simulink model "PMSM_braking_regen_and_Eddy_current_using_ABS"  (R2023a)
settings: Solver=VariableStepAuto  StartTime=0.0  StopTime=20  MaxStep=1  RelTol=1e-3
libraries: spsControlledVoltageSourceLib x3, spsVoltageMeasurementLib x3, simulink x2, spsPermanentMagnetSynchronousMachineLib x1, spsThreePhaseSineGeneratorLib x1, sps_lib x1
settings Model: Creator=siddh  LastModifiedBy=siddh

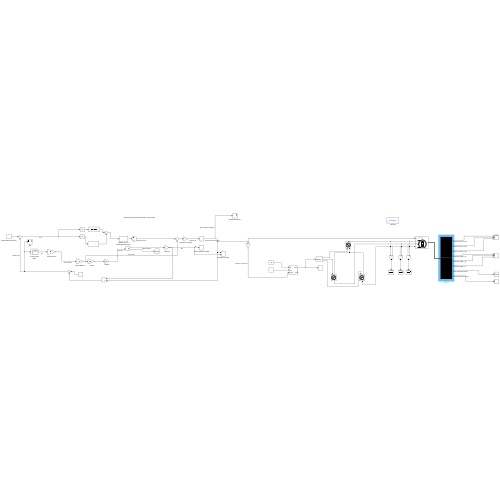
[thumbnail: Simulink's stored preview of the top-level diagram]
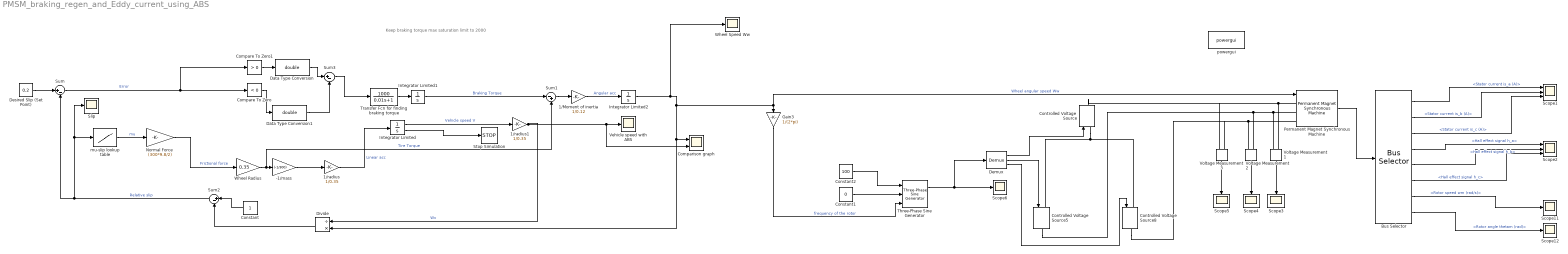
== system PMSM_braking_regen_and_Eddy_current_using_ABS ==
  note: Keep braking torque max saturation limit to 2000
  -1/mass : Gain  Gain=(-1/300)
  1/Moment of inertia : Gain  Gain=1/0.12
  1/radius : Gain  Gain=1/0.35
  1/radius1 : Gain  Gain=1/0.35
  Bus Selector : BusSelector  OutputSignals=Stator current is_a (A),Stator current is_b (A),Stator current is_c (A),Hall effect signal h_a,Hall effect signal h_b,Hall effect signal h_c,Rotor speed wm (rad/s),Rotor angle thetam (rad)
  Compare To Zero : simulink/Logic and Bit Operations/Compare To Zero  relop=<  OutDataTypeStr=boolean
  Compare To Zero1 : simulink/Logic and Bit Operations/Compare To Zero  relop=>  OutDataTypeStr=boolean
  Comparison graph : Scope  NumInputPorts=2
  Constant : Constant
  Constant1 : Constant  Value=0
  Constant2 : Constant  Value=100
  Controlled Voltage Source : spsControlledVoltageSourceLib/Controlled Voltage Source  Initialize=on  Source_Type=AC  Amplitude=100  Phase=0  Frequency=0  Measurements=None
  Controlled Voltage Source5 : spsControlledVoltageSourceLib/Controlled Voltage Source  Initialize=on  Source_Type=AC  Amplitude=0  Phase=0  Frequency=0  Measurements=None
  Controlled Voltage Source8 : spsControlledVoltageSourceLib/Controlled Voltage Source  Initialize=on  Source_Type=AC  Amplitude=0  Phase=0  Frequency=0  Measurements=None
  Data Type Conversion : DataTypeConversion  OutDataTypeStr=double  SaturateOnIntegerOverflow=off
  Data Type Conversion1 : DataTypeConversion  OutDataTypeStr=double  SaturateOnIntegerOverflow=off
  Demux : Demux  Outputs=3
      settings: DisplayOption=none
  "Desired Slip (Set Point) " : Constant  Value=0.2
  Divide : Product  Inputs=/*
  Gain3 : Gain  Gain=1/(2*pi)
  Integrator Limited : Integrator  InitialCondition=30  LimitOutput=on  UpperSaturationLimit=500  LowerSaturationLimit=0  ShowSaturationPort=on
  Integrator Limited1 : Integrator  LimitOutput=on  UpperSaturationLimit=2000  LowerSaturationLimit=0
  Integrator Limited2 : Integrator  InitialCondition=30/0.35  LimitOutput=on  UpperSaturationLimit=500  LowerSaturationLimit=0
  Normal Force : Gain  Gain=(300*9.8/2)
  Permanent Magnet Synchronous Machine : spsPermanentMagnetSynchronousMachineLib/Permanent Magnet Synchronous Machine  NbPhases=3  FluxDistribution=Sinusoidal  RotorType=Round  MechanicalLoad=Speed w  PresetModel=No  ShowDetailedParameters=on  MeasurementBus=off  Resistance=18.7  Inductance=8.5e-3  dqInductances=[8.5e-3,8.5e-3]  La=0.02682  MachineConstant=Flux linkage established by magnets (V.s)  Flux=0.1716  VoltageCst=62.2496  TorqueCst=0.5148  Flat=120  Mechanical=[2.26e-05 1.349e-05 2 0]  PolePairs=2  InitialConditions=[0,0, 0,0]  InitialConditions5ph=[0 0 0 0 0 0]  RefAngle=90 degrees behind phase A axis (modified Park)  IterativeDiscreteModel=Trapezoidal non iterative  TsBlock=-1  TsPowergui=0
  Scope1 : Scope  NumInputPorts=3
  Scope{3..6,11..12} (6 alike) : Scope
  Scope2 : Scope  NumInputPorts=3
  "Slip " : Scope
  Stop Simulation : Stop
  Sum : Sum  Inputs=|+-
  Sum1 : Sum  Inputs=|-+
  Sum2 : Sum  Inputs=|+-
  Sum3 : Sum  Inputs=|+-
  Three-Phase Sine Generator : spsThreePhaseSineGeneratorLib/Three-Phase Sine Generator  Ts=0
      settings: LibrarySourceBlock=|
      | sps_lib/Sources/Signal Generator Sources/Three-Phase
      | Sine Generator
  Transfer Fcn for finding braking torque : TransferFcn  Numerator=[1000]  Denominator=[0.01 1]
  Vehicle speed with ABS : Scope
  Voltage Measurement1 : spsVoltageMeasurementLib/Voltage Measurement  PhasorSimulation=off  OutputType=Complex  PSBequivalent=0
  Voltage Measurement2 : spsVoltageMeasurementLib/Voltage Measurement  PhasorSimulation=off  OutputType=Complex  PSBequivalent=0
  Voltage Measurement3 : spsVoltageMeasurementLib/Voltage Measurement  PhasorSimulation=off  OutputType=Complex  PSBequivalent=0
  Wheel Radius : Gain  Gain=0.35
  Wheel Speed Ww : Scope
  mu-slip lookup table : Lookup_n-D  NumberOfTableDimensions=1  BreakpointsForDimension1=[0,0.05,0.1,0.15,0.2,0.25,0.3,0.35,0.4,0.45,0.5,0.55,0.60,0.65,0.70,0.75,0.80,0.85,0.90,0.95,1]  Table=[0,0.4,0.8,0.97,1,0.98,0.96,0.94,0.92,0.9,0.88,0.855,0.83,0.81,0.79,0.77,0.75,0.73,0.72,0.71,0.7]  InternalRulePriority=Speed  RndMeth=Simplest
  powergui : sps_lib/powergui  Priority=1  SimulationMode=Continuous  SampleTime=50e-6  frequency=60  Iterations=50  frequencyindice=0  Pbase=100e6  ErrMax=1e-4  UnitsV=kV  UnitsW=MW  buscounter=0  FunctionMessages=off  echomessages=off  EnableUseOfTLC=off  CurrentSourceSwitches=off  DisableSnubberDevices=off  DisableRonSwitches=off  DisableVfSwitches=off  DisplayEquations=off  AutomaticDiscreteSolvers=off  SolverType=Tustin/Backward Euler (TBE)  Interpol=off  ExternalGateDelay=off  methode=off  Ts=100  x0status=blocks  SPID=on  SwTol=0  HookPort=off  NonlinearTolerance=1e-4  nMaxIteration=100  ContinueOnMaxIteration=off  RestoreLinks=warning  ResistiveCurrentMeasurement=off  Frange=[0:2:500]  Ylog=off  Xlog=on  ShowGrid=off  save=off  variable=ZData  structure=0  ZoomFFT=off  StartTime=0.0  cycles=1  DisplayStyle=1  fundamental=60  FreqAxis=off  MaxFrequency=1000  frequencyindicesteady=1  RmsSteady=1  display=off
  wires:
  Voltage Measurement3/1 -> Scope5/1
  Voltage Measurement1/1 -> Scope3/1
  Bus Selector/8 -> Scope12/1  "<Rotor angle thetam (rad)>"
  Bus Selector/7 -> Scope11/1  "<Rotor speed wm (rad/s)>"
  Bus Selector/1 -> Scope1/1  "<Stator current is_a (A)>"
  Bus Selector/2 -> Scope1/2  "<Stator current is_b (A)>"
  Bus Selector/3 -> Scope1/3  "<Stator current is_c (A)>"
  Bus Selector/5 -> Scope2/2  "<Hall effect signal h_b>"
  Bus Selector/4 -> Scope2/1  "<Hall effect signal h_a>"
  Bus Selector/6 -> Scope2/3  "<Hall effect signal h_c>"
  Voltage Measurement2/1 -> Scope4/1
  Permanent Magnet Synchronous Machine/1 -> Bus Selector/1
  Constant2/1 -> Three-Phase Sine Generator/1
  Constant1/1 -> Three-Phase Sine Generator/2
  Gain3/1 -> Three-Phase Sine Generator/3  "frequency of the rotor"
  Three-Phase Sine Generator/1 -> Demux/1, Scope6/1
  Demux/1 -> Controlled Voltage Source/1
  Demux/2 -> Controlled Voltage Source5/1
  Demux/3 -> Controlled Voltage Source8/1
  1/radius1/1 -> Divide/1, Comparison graph/2, Vehicle speed with ABS/1  "Wv"
  Compare To Zero1/1 -> Data Type Conversion/1
  Compare To Zero/1 -> Data Type Conversion1/1
  Data Type Conversion/1 -> Sum3/1
  Sum3/1 -> Transfer Fcn for finding braking torque/1
  Integrator Limited2/1 -> Permanent Magnet Synchronous Machine/1, Gain3/1, Divide/2, Comparison graph/1, Wheel Speed Ww/1  "Wheel angular speed Ww"
  Sum1/1 -> 1/Moment of inertia/1
  Integrator Limited1/1 -> Sum1/1  "Braking Torque"
  Data Type Conversion1/1 -> Sum3/2
  Constant/1 -> Sum2/1
  1/Moment of inertia/1 -> Integrator Limited2/1  "Angular acc"
  Integrator Limited/2 -> Stop Simulation/1
  "Desired Slip (Set Point) "/1 -> Sum/1
  1/radius/1 -> Integrator Limited/1  "Linear acc"
  Sum2/1 -> "Slip "/1, mu-slip lookup table/1, Sum/2  "Relative slip"
  Normal Force/1 -> Wheel Radius/1  "Frictional force"
  -1/mass/1 -> 1/radius/1
  Divide/1 -> Sum2/2
  mu-slip lookup table/1 -> Normal Force/1  "mu"
  Sum/1 -> Compare To Zero/1, Compare To Zero1/1  "Error"
  Transfer Fcn for finding braking torque/1 -> Integrator Limited1/1
  Wheel Radius/1 -> Sum1/2, -1/mass/1  "Tire Torque"
  Integrator Limited/1 -> 1/radius1/1  "Vehicle speed V"
  connections:
  Voltage Measurement2/LConn2 -- Controlled Voltage Source8/RConn1 -- Voltage Measurement3/LConn1 -- Permanent Magnet Synchronous Machine/LConn3
  Voltage Measurement1/LConn1 -- Controlled Voltage Source/RConn1 -- Voltage Measurement3/LConn2 -- Permanent Magnet Synchronous Machine/LConn1
  Voltage Measurement2/LConn1 -- Permanent Magnet Synchronous Machine/LConn2 -- Voltage Measurement1/LConn2 -- Controlled Voltage Source5/RConn1
  Controlled Voltage Source/LConn1 -- Controlled Voltage Source5/LConn1 -- Controlled Voltage Source8/LConn1
